simulink model "F16ASYM_Controlled"  (R2015a)
settings: Solver=ode3  SolverMode=SingleTasking  StartTime=0.0  StopTime=inf  FixedStep=T_sim  RelTol=1e-3
InitFcn:
  | load('NN_c_weights_Last_stable.mat')
StopFcn:
  | Final_results
values from neighbouring files (symbols this model uses):
  a1 = fitresult.p1    [Stall_protection.m]
  alpha_map_eval = ones(size(M_eval))*NaN    [Auto_trim_aid.m]    (also in Autotrim_maps.mat = [nan nan 0.277598136245 0.119432432992 0.0579479097061 0.027)
  beta_map_eval = ones(size(M_eval))*NaN    [Auto_trim_aid.m]    (also in Autotrim_maps.mat = [nan nan -0.00151549403324 0.00117807579006 -0.0052086799721)
  C_L_0 = fitresult.p2    [Stall_protection.m]
  G_eval = NaN*ones(size(M_sq,2),size(H_sq,2))    [Stall_protection.m]
  H_sq = unique(sort(H_sq))    [Stall_protection.m]
  H_sq_autotrim = min( F_envelope.H_1g):2000:max(F_envelope.H_1g)    [Auto_trim_aid.m]    (also in Autotrim_maps.mat = [0 2000 4000 6000 8000 10000 12000 14000 16000 18000])
  K_b_q_extrap_ACC = K_b_q_extrap    [RUN_ME.m]
  K_b_q_extrap_AoA = K_b_q_extrap    [RUN_ME.m]
  M_sq = unique(sort(M_sq))    [Stall_protection.m]
  M_sq_autotrim = 0:0.1:max(F_envelope.M_1g)    [Auto_trim_aid.m]    (also in Autotrim_maps.mat = [0 0.1 0.2 0.3 0.4 0.5 0.6 0.7 0.8 0.9 1 1.1 ... (21 element)
  T_sim = 0.02    [RUN_ME.m]
  tau_q_extrap_ACC = tau_q_extrap    [RUN_ME.m]
  tau_q_extrap_AoA = tau_q_extrap    [RUN_ME.m]
  velocity = M_eval(I,J)*a    [Auto_trim_aid.m]
undefined symbols (not defined in the file or in its folder): ACCEL, B, Earth, fi_flag_Simulink, GYRO, H_sq_sche, k_B, K_b_ACC_extrap, K_b_AoA_extrap, latitude, longitude, m, m_B, M_sq_sche, Model_used_flag, rad, s, sigbuilder_block, Stall_curve, tau_ACC_extrap, tau_AoA_extrap, Theta_1_roll_last, Theta_2_roll_last, Theta_3_roll_last, trim_control, trim_state, trim_throttle, V_Comp_A_w_z_last, V_Comp_last, V_Comp_last_ONE, V_long_lastA_w_z, V_long_lastAoA, V_roll_last, V_roll_lastMOD, V_yaw_last, W_Comp_A_w_z_last, W_Comp_last, W_long_lastA_w_z, W_long_lastAoA, W_roll_last, W_roll_lastMOD, W_yaw_last, WGS84
libraries: Adaptive_FaultTolerantControl x57, dspsigops x37, F16_Actuator_Library x14, commnoisgen2 x13, simulink x11, simulink_extras x10, dsparch4 x6, aerolibatmos2 x6, aerolibtransform2 x6, aerolibfltsims x3, dspvision x3, dspsnks4 x3
(part 6 of 14)

== system F16ASYM_Controlled/Primary Controller/P cont + adaptive Crossed NN + AWU+Lim ONELAYER/Physical limitation ==
  note: Converto to Angular accelerations
  v comm : Inport
  all meas : Inport  Port=2
  Ang Accel : MATLAB Function
  Bus Selector : BusSelector  OutputSignals=signal1.Alt meas (m),signal1.V_TAS (m/s),signal1.AoA meas (rad),signal1.SS meas (rad),signal1.omega_b meas (rad/s),signal1.Throttle_meas
  Bus Selector1 : BusSelector  OutputSignals=signal2.q (Pa),signal1.omega_b meas (rad/s)
  Demux : Demux  Outputs=3
  Display : Display
  Display1 : Display
  Display2 : Display
  Divide : Product  Inputs=**
  Divide1 : Product  Inputs=**
  Gain : Gain  Gain=-1
  Gain1 : Gain
  Mom coefficients that can be reached : MATLABFcn  MATLABFcn=Moms_Coeff_estimator  OutputDimensions=3  OutputSignalType=real
  Moments : Subsystem
  Mux : Mux  Inputs=3
  Mux1 : Mux  Inputs=7
  Saturation Dynamic : simulink/Discontinuities/Saturation Dynamic  OutMin=[]  OutMax=[]  OutDataTypeStr=Inherit: Same as second input  OutDataType=fixdt(1, 16)  OutScaling=2^-10  DoSatur=off
  Sign : Signum
  Sign1 : Signum
  max deflections estimator : MATLAB Function  TreatAsAtomicUnit=on
  v limted : Outport
  wires:
  max deflections estimator/1(max_defl) -> Mux1/7
  Mux1/1 -> Mom coefficients that can be reached/1
  Bus Selector/5 -> Mux1/5  "<omega_b meas (rad/s)>"
  Bus Selector/1 -> Mux1/1  "<Alt meas (m)>"
  Bus Selector/2 -> Mux1/2  "<V_TAS (m/s)>"
  Bus Selector/3 -> Mux1/3  "<AoA meas (rad)>"
  Bus Selector/4 -> Mux1/4  "<SS meas (rad)>"
  Bus Selector/6 -> Mux1/6  "<Throttle_meas>"
  Ang Accel/2(q_dot) -> Mux/2
  Ang Accel/3(r_dot) -> Mux/3
  Ang Accel/1(p_dot) -> Mux/1
  Bus Selector1/2 -> Ang Accel/4(omega_b)  "<omega_b meas (rad/s)>"
  Moments/3(N) -> Ang Accel/3(N)
  Moments/2(M) -> Ang Accel/2(M)
  Moments/1(L) -> Ang Accel/1(L)
  Bus Selector1/1 -> Moments/4(q)  "<q (Pa)>"
  Demux/3 -> Moments/3(C_N)
  Demux/2 -> Moments/2(C_M)
  Demux/1 -> Moments/1(C_L)
  Mom coefficients that can be reached/1 -> Demux/1
  all meas/1 -> Bus Selector/1, Bus Selector1/1
  Mux/1 -> Gain1/1
  v comm/1 -> Saturation Dynamic/2, Display1/1, max deflections estimator/1(v_comm)
  Saturation Dynamic/1 -> Display/1, v limted/1
  Sign/1 -> Divide/1
  Gain1/1 -> Divide/2, Divide1/1, Sign1/1, Display2/1, Sign/1
  Sign1/1 -> Gain/1
  Divide/1 -> Saturation Dynamic/1
  Gain/1 -> Divide1/2
  Divide1/1 -> Saturation Dynamic/3

== system F16ASYM_Controlled/Primary Controller/P cont + adaptive Crossed NN + AWU+Lim ONELAYER/Sigmoid  ==
  In : Inport
  Display : Display
  Fcn1 : Fcn  Commented=on  Expr=2.0 ./ (1.0 + exp(-u(4)*u(1:3)))-1
  MATLAB Function : MATLAB Function  TreatAsAtomicUnit=on
  a : Constant  Value=a
  Out : Outport
  wires:
  MATLAB Function/1(y) -> Display/1, Out/1
  In/1 -> MATLAB Function/1(u)
  a/1 -> MATLAB Function/2(a)

== system F16ASYM_Controlled/Primary Controller/P controller/Body Rates Controller ==
  p_ref : Inport
  q_ref : Inport  Port=2
  r_ref : Inport  Port=3
  All_meas : Inport  Port=4
  Bus Creator : BusCreator
  Bus Creator1 : BusCreator
  Bus Creator2 : BusCreator
  Bus Selector : BusSelector  OutputSignals=signal1.omega_b meas (rad/s)
  Display1 : Display
  Mux : Mux  Inputs=3
  Ref Model and P Controller p : Adaptive_FaultTolerantControl/Ref Model and P Controller  tau=0.1  y_i=trim_state(10)  K_f=1  K_b=7
  Ref Model and P Controller q : Adaptive_FaultTolerantControl/Ref Model and P Controller  tau=0.08  y_i=trim_state(11)  K_f=1  K_b=3.5
  Ref Model and P Controller r : Adaptive_FaultTolerantControl/Ref Model and P Controller  tau=0.08  y_i=trim_state(12)  K_f=1  K_b=4
  Selector : Selector  InputPortWidth=3
  Selector1 : Selector  InputPortWidth=3  Indices=2
  Selector2 : Selector  InputPortWidth=3  Indices=3
  Sum : Sum  Inputs=+-|
  Sum1 : Sum  Inputs=+-|
  Sum2 : Sum  Inputs=+-|
  Terminator1 : Terminator
  Terminator2 : Terminator
  Terminator3 : Terminator
  Angular acc des (rad/s^2) : Outport
  wires:
  Ref Model and P Controller r/5 -> Bus Creator2/4  "K_b_r"
  Ref Model and P Controller r/4 -> Sum2/2
  Sum2/1 -> Bus Creator2/3  "p_err"
  Ref Model and P Controller r/3 -> Bus Creator2/2, Sum2/1  "p_sf"
  Ref Model and P Controller r/2 -> Bus Creator2/1  "p_sf_dot"
  Ref Model and P Controller q/5 -> Bus Creator1/4  "K_b_q"
  Ref Model and P Controller q/4 -> Sum1/2
  Sum1/1 -> Bus Creator1/3  "p_err"
  Ref Model and P Controller q/3 -> Bus Creator1/2, Sum1/1  "p_sf"
  Ref Model and P Controller q/2 -> Bus Creator1/1  "p_sf_dot"
  Ref Model and P Controller p/5 -> Bus Creator/4  "K_b_p"
  Ref Model and P Controller p/4 -> Sum/2
  Selector2/1 -> Ref Model and P Controller r/2
  Bus Creator2/1 -> Terminator3/1
  Bus Creator1/1 -> Terminator1/1
  Bus Creator/1 -> Terminator2/1
  Sum/1 -> Bus Creator/3, Display1/1  "p_err"
  Ref Model and P Controller p/3 -> Bus Creator/2, Sum/1  "p_sf"
  Ref Model and P Controller p/2 -> Bus Creator/1  "p_sf_dot"
  Ref Model and P Controller r/1 -> Mux/3
  Ref Model and P Controller q/1 -> Mux/2
  r_ref/1 -> Ref Model and P Controller r/1
  Selector1/1 -> Ref Model and P Controller q/2
  q_ref/1 -> Ref Model and P Controller q/1
  Mux/1 -> Angular acc des (rad/s^2)/1
  Ref Model and P Controller p/1 -> Mux/1
  Selector/1 -> Ref Model and P Controller p/2
  p_ref/1 -> Ref Model and P Controller p/1
  Bus Selector/1 -> Selector2/1, Selector1/1, Selector/1  "<omega_b meas (rad/s)>"
  All_meas/1 -> Bus Selector/1

== system F16ASYM_Controlled/Primary Controller/P controller/Lat_dir Dyn Inversion: beta_dot->r_c ==
  beta_dot_c : Inport
  All_meas : Inport  Port=2
  A_w_y : Selector  InputPortWidth=3  Indices=2
  Bus Selector : BusSelector  OutputSignals=signal1.AoA meas (rad),signal1.omega_b meas (rad/s),signal1.V_TAS (m/s),signal2.A_w_CG
  Divide1 : Product  Inputs=**
  Divide3 : Product  Inputs=**
  Divide4 : Product  Inputs=/*
  Divide5 : Product  Inputs=*/
  Selector : Selector  InputPortWidth=3
  Trigonometric Function : Trigonometry  Operator=cos
  Trigonometric Function3 : Trigonometry  Operator=tan
  "q_c " : Sum  Inputs=-++
  r_c : Outport
  wires:
  Selector/1 -> Divide1/2
  Trigonometric Function3/1 -> Divide1/1
  beta_dot_c/1 -> Divide5/1
  Divide5/1 -> "q_c "/1
  Trigonometric Function/1 -> Divide5/2, Divide3/1
  Bus Selector/3 -> Divide3/2  "<V_TAS (m/s)>"
  Divide4/1 -> "q_c "/3
  Bus Selector/4 -> A_w_y/1  "<A_w_CG>"
  All_meas/1 -> Bus Selector/1
  A_w_y/1 -> Divide4/2
  Divide3/1 -> Divide4/1
  Divide1/1 -> "q_c "/2
  Bus Selector/2 -> Selector/1  "<omega_b meas (rad/s)>"
  Bus Selector/1 -> Trigonometric Function3/1, Trigonometric Function/1  "<AoA meas (rad)>"
  "q_c "/1 -> r_c/1

== system F16ASYM_Controlled/Primary Controller/P controller/Long Dyn Inversion: alpha_dot ->q ==
  alpha_dot_c : Inport
  All_meas : Inport  Port=2
  Completed : Subsystem
  Manual Switch : ManualSwitch
  Simplified : Subsystem
  q_c : Outport
  wires:
  Manual Switch/1 -> q_c/1
  Simplified/1(q_c) -> Manual Switch/2
  Completed/1(q_c) -> Manual Switch/1
  All_meas/1 -> Completed/2(All_meas), Simplified/2(All_meas)
  alpha_dot_c/1 -> Completed/1(alpha_dot_c), Simplified/1(alpha_dot_c)

== system F16ASYM_Controlled/Primary Controller/P controller/Longitudinal Controller: AoA or A_w_z ==
  A_w_z des : Inport
  AoA des (rad) : Inport  Port=2
  Anti-windup A_w_z : Inport  Port=3
  Anti-windup AoA : Inport  Port=4
  All meas : Inport  Port=5
  Longitudinal controller in A_w_z : Subsystem  VariantControl=Controller of A_w_z
  Longitudinal controller in AoA : Subsystem  VariantControl=Controller of AoA
  A_chanel vars : Outport
  alpha_chanel vars : Outport  Port=2
  alpha_dot_c : Outport  Port=3

== system F16ASYM_Controlled/Primary Controller/P controller + adaptive Crossed NN/Body Rates Controller ==
  p_ref : Inport
  q_ref : Inport  Port=2
  r_ref : Inport  Port=3
  All_meas : Inport  Port=4
  Bus Creator : BusCreator
  Bus Creator1 : BusCreator
  Bus Creator2 : BusCreator
  Bus Selector : BusSelector  OutputSignals=signal1.omega_b meas (rad/s)
  Display1 : Display
  Mux : Mux  Inputs=3
  Ref Model and P Controller p : Adaptive_FaultTolerantControl/Ref Model and P Controller  tau=0.1  y_i=trim_state(10)  K_f=1  K_b=7
  Ref Model and P Controller q : Adaptive_FaultTolerantControl/Ref Model and P Controller  tau=0.25  y_i=trim_state(11)  K_f=1  K_b=7
  Ref Model and P Controller r : Adaptive_FaultTolerantControl/Ref Model and P Controller  tau=0.2  y_i=trim_state(12)  K_f=1  K_b=4
  Selector : Selector  InputPortWidth=3
  Selector1 : Selector  InputPortWidth=3  Indices=2
  Selector2 : Selector  InputPortWidth=3  Indices=3
  Sum : Sum  Inputs=+-|
  Sum1 : Sum  Inputs=+-|
  Sum2 : Sum  Inputs=+-|
  q_chanel vars : Outport
  p_chanel vars : Outport  Port=2
  r_chanel vars : Outport  Port=3
  Angular acc des (rad/s^2) : Outport  Port=4
  wires:
  Ref Model and P Controller r/5 -> Bus Creator2/4  "K_b_r"
  Ref Model and P Controller r/4 -> Sum2/2
  Sum2/1 -> Bus Creator2/3  "r_err"
  Ref Model and P Controller r/3 -> Bus Creator2/2, Sum2/1  "r_sf"
  Ref Model and P Controller r/2 -> Bus Creator2/1  "r_sf_dot"
  Ref Model and P Controller q/5 -> Bus Creator1/4  "K_b_q"
  Ref Model and P Controller q/4 -> Sum1/2
  Sum1/1 -> Bus Creator1/3  "q_err"
  Ref Model and P Controller q/3 -> Bus Creator1/2, Sum1/1  "q_sf"
  Ref Model and P Controller q/2 -> Bus Creator1/1  "q_sf_dot"
  Ref Model and P Controller p/5 -> Bus Creator/4  "K_b_p"
  Ref Model and P Controller p/4 -> Sum/2
  Selector2/1 -> Ref Model and P Controller r/2
  Bus Creator2/1 -> r_chanel vars/1
  Bus Creator1/1 -> q_chanel vars/1
  Bus Creator/1 -> p_chanel vars/1
  Sum/1 -> Bus Creator/3, Display1/1  "p_err"
  Ref Model and P Controller p/3 -> Bus Creator/2, Sum/1  "p_sf"
  Ref Model and P Controller p/2 -> Bus Creator/1  "p_sf_dot"
  Ref Model and P Controller r/1 -> Mux/3
  Ref Model and P Controller q/1 -> Mux/2
  r_ref/1 -> Ref Model and P Controller r/1
  Selector1/1 -> Ref Model and P Controller q/2
  q_ref/1 -> Ref Model and P Controller q/1
  Mux/1 -> Angular acc des (rad/s^2)/1
  Ref Model and P Controller p/1 -> Mux/1
  Selector/1 -> Ref Model and P Controller p/2
  p_ref/1 -> Ref Model and P Controller p/1
  Bus Selector/1 -> Selector2/1, Selector1/1, Selector/1  "<omega_b meas (rad/s)>"
  All_meas/1 -> Bus Selector/1

== system F16ASYM_Controlled/Primary Controller/P controller + adaptive Crossed NN/Complete crossed On-line (adaptive) multi-layer NN ==
  v_ad^ prev : Inport
  All_meas : Inport  Port=2
  NN variables : Inport  Port=3
  Complete crossed On-line (adaptive) multi-layer NN: A_w_z : Subsystem  VariantControl=NN on A_w_z
  Complete crossed On-line (adaptive) multi-layer NN: AoA : Subsystem  VariantControl=NN on AoA
  v_ad^ : Outport

== system F16ASYM_Controlled/Primary Controller/P controller + adaptive Crossed NN/Lat_dir Dyn Inversion: beta_dot->r_c ==
  beta_dot_c : Inport
  All_meas : Inport  Port=2
  A_w_y : Selector  InputPortWidth=3  Indices=2
  Bus Selector : BusSelector  OutputSignals=signal1.AoA meas (rad),signal1.omega_b meas (rad/s),signal1.V_TAS (m/s),signal2.A_w_CG
  Divide1 : Product  Inputs=**
  Divide3 : Product  Inputs=**
  Divide4 : Product  Inputs=/*
  Divide5 : Product  Inputs=*/
  Selector : Selector  InputPortWidth=3
  Trigonometric Function : Trigonometry  Operator=cos
  Trigonometric Function3 : Trigonometry  Operator=tan
  "q_c " : Sum  Inputs=-++
  r_c : Outport
  wires:
  Selector/1 -> Divide1/2
  Trigonometric Function3/1 -> Divide1/1
  beta_dot_c/1 -> Divide5/1
  Divide5/1 -> "q_c "/1
  Trigonometric Function/1 -> Divide5/2, Divide3/1
  Bus Selector/3 -> Divide3/2  "<V_TAS (m/s)>"
  Divide4/1 -> "q_c "/3
  Bus Selector/4 -> A_w_y/1  "<A_w_CG>"
  All_meas/1 -> Bus Selector/1
  A_w_y/1 -> Divide4/2
  Divide3/1 -> Divide4/1
  Divide1/1 -> "q_c "/2
  Bus Selector/2 -> Selector/1  "<omega_b meas (rad/s)>"
  Bus Selector/1 -> Trigonometric Function3/1, Trigonometric Function/1  "<AoA meas (rad)>"
  "q_c "/1 -> r_c/1

== system F16ASYM_Controlled/Primary Controller/P controller + adaptive Crossed NN/Long Dyn Inversion: alpha_dot ->q ==
  alpha_dot_c : Inport
  All_meas : Inport  Port=2
  Completed : Subsystem
  Manual Switch : ManualSwitch
  Simplified : Subsystem
  q_c : Outport
  wires:
  Manual Switch/1 -> q_c/1
  Simplified/1(q_c) -> Manual Switch/2
  Completed/1(q_c) -> Manual Switch/1
  All_meas/1 -> Completed/2(All_meas), Simplified/2(All_meas)
  alpha_dot_c/1 -> Completed/1(alpha_dot_c), Simplified/1(alpha_dot_c)

== system F16ASYM_Controlled/Primary Controller/P controller + adaptive Crossed NN/Longitudinal Controller: AoA or A_w_z ==
  A_w_z des : Inport
  AoA des (rad) : Inport  Port=2
  Anti-windup A_w_z : Inport  Port=3
  Anti-windup AoA : Inport  Port=4
  All meas : Inport  Port=5
  Longitudinal controller in A_w_z : Subsystem  VariantControl=Controller of A_w_z
  Longitudinal controller in AoA : Subsystem  VariantControl=Controller of AoA
  A_chanel vars : Outport
  alpha_chanel vars : Outport  Port=2
  alpha_dot_c : Outport  Port=3

== system F16ASYM_Controlled/Primary Controller/P controller + adaptive Crossed NN/Sigmoid  ==
  In : Inport
  Display : Display
  Fcn1 : Fcn  Commented=on  Expr=2.0 ./ (1.0 + exp(-u(4)*u(1:3)))-1
  MATLAB Function : MATLAB Function  TreatAsAtomicUnit=on
  a : Constant  Value=a
  Out : Outport
  wires:
  a/1 -> MATLAB Function/2(a)
  In/1 -> MATLAB Function/1(u)
  MATLAB Function/1(y) -> Out/1, Display/1

== system F16ASYM_Controlled/Primary Controller/P controller + adaptive Isolated NN/Body Rates Controller ==
  p_ref : Inport
  q_ref : Inport  Port=2
  r_ref : Inport  Port=3
  All_meas : Inport  Port=4
  Bus Creator : BusCreator
  Bus Creator1 : BusCreator
  Bus Creator2 : BusCreator
  Bus Selector : BusSelector  OutputSignals=signal1.omega_b meas (rad/s)
  Display1 : Display
  Mux : Mux  Inputs=3
  Ref Model and P Controller p : Adaptive_FaultTolerantControl/Ref Model and P Controller  tau=0.1  y_i=trim_state(10)  K_f=1  K_b=7
  Ref Model and P Controller q : Adaptive_FaultTolerantControl/Ref Model and P Controller  tau=0.25  y_i=trim_state(11)  K_f=1  K_b=8
  Ref Model and P Controller r : Adaptive_FaultTolerantControl/Ref Model and P Controller  tau=0.2  y_i=trim_state(12)  K_f=1  K_b=4
  Selector : Selector  InputPortWidth=3
  Selector1 : Selector  InputPortWidth=3  Indices=2
  Selector2 : Selector  InputPortWidth=3  Indices=3
  Sum : Sum  Inputs=+-|
  Sum1 : Sum  Inputs=+-|
  Sum2 : Sum  Inputs=+-|
  q_chanel vars : Outport
  p_chanel vars : Outport  Port=2
  r_chanel vars : Outport  Port=3
  Angular acc des (rad/s^2) : Outport  Port=4
  wires:
  All_meas/1 -> Bus Selector/1
  Bus Selector/1 -> Selector/1, Selector1/1, Selector2/1  "<omega_b meas (rad/s)>"
  p_ref/1 -> Ref Model and P Controller p/1
  Selector/1 -> Ref Model and P Controller p/2
  Ref Model and P Controller p/1 -> Mux/1
  Mux/1 -> Angular acc des (rad/s^2)/1
  q_ref/1 -> Ref Model and P Controller q/1
  Selector1/1 -> Ref Model and P Controller q/2
  r_ref/1 -> Ref Model and P Controller r/1
  Ref Model and P Controller q/1 -> Mux/2
  Ref Model and P Controller r/1 -> Mux/3
  Ref Model and P Controller p/2 -> Bus Creator/1  "p_sf_dot"
  Ref Model and P Controller p/3 -> Sum/1, Bus Creator/2  "p_sf"
  Sum/1 -> Display1/1, Bus Creator/3  "p_err"
  Bus Creator/1 -> p_chanel vars/1
  Bus Creator1/1 -> q_chanel vars/1
  Bus Creator2/1 -> r_chanel vars/1
  Selector2/1 -> Ref Model and P Controller r/2
  Ref Model and P Controller p/4 -> Sum/2
  Ref Model and P Controller p/5 -> Bus Creator/4  "K_b_p"
  Ref Model and P Controller q/2 -> Bus Creator1/1  "q_sf_dot"
  Ref Model and P Controller q/3 -> Sum1/1, Bus Creator1/2  "q_sf"
  Sum1/1 -> Bus Creator1/3  "q_err"
  Ref Model and P Controller q/4 -> Sum1/2
  Ref Model and P Controller q/5 -> Bus Creator1/4  "K_b_q"
  Ref Model and P Controller r/2 -> Bus Creator2/1  "r_sf_dot"
  Ref Model and P Controller r/3 -> Sum2/1, Bus Creator2/2  "r_sf"
  Sum2/1 -> Bus Creator2/3  "r_err"
  Ref Model and P Controller r/4 -> Sum2/2
  Ref Model and P Controller r/5 -> Bus Creator2/4  "K_b_r"

== system F16ASYM_Controlled/Primary Controller/P controller + adaptive Isolated NN/Lat_dir Dyn Inversion: beta_dot->r_c ==
  beta_dot_c : Inport
  All_meas : Inport  Port=2
  A_w_y : Selector  InputPortWidth=3  Indices=2
  Bus Selector : BusSelector  OutputSignals=signal1.AoA meas (rad),signal1.omega_b meas (rad/s),signal1.V_TAS (m/s),signal2.A_w_CG
  Divide1 : Product  Inputs=**
  Divide3 : Product  Inputs=**
  Divide4 : Product  Inputs=/*
  Divide5 : Product  Inputs=*/
  Selector : Selector  InputPortWidth=3
  Trigonometric Function : Trigonometry  Operator=cos
  Trigonometric Function3 : Trigonometry  Operator=tan
  "q_c " : Sum  Inputs=-++
  r_c : Outport
  wires:
  "q_c "/1 -> r_c/1
  Bus Selector/1 -> Trigonometric Function/1, Trigonometric Function3/1  "<AoA meas (rad)>"
  Bus Selector/2 -> Selector/1  "<omega_b meas (rad/s)>"
  Divide1/1 -> "q_c "/2
  Divide3/1 -> Divide4/1
  A_w_y/1 -> Divide4/2
  All_meas/1 -> Bus Selector/1
  Bus Selector/4 -> A_w_y/1  "<A_w_CG>"
  Divide4/1 -> "q_c "/3
  Bus Selector/3 -> Divide3/2  "<V_TAS (m/s)>"
  Trigonometric Function/1 -> Divide3/1, Divide5/2
  Divide5/1 -> "q_c "/1
  beta_dot_c/1 -> Divide5/1
  Trigonometric Function3/1 -> Divide1/1
  Selector/1 -> Divide1/2

== system F16ASYM_Controlled/Primary Controller/P controller + adaptive Isolated NN/Long Dyn Inversion: alpha_dot ->q ==
  alpha_dot_c : Inport
  All_meas : Inport  Port=2
  Completed : Subsystem
  Manual Switch : ManualSwitch
  Simplified : Subsystem
  q_c : Outport
  wires:
  alpha_dot_c/1 -> Simplified/1(alpha_dot_c), Completed/1(alpha_dot_c)
  All_meas/1 -> Simplified/2(All_meas), Completed/2(All_meas)
  Completed/1(q_c) -> Manual Switch/1
  Simplified/1(q_c) -> Manual Switch/2
  Manual Switch/1 -> q_c/1

== system F16ASYM_Controlled/Primary Controller/P controller + adaptive Isolated NN/Longitudinal Controller: AoA or A_w_z ==
  A_w_z des : Inport
  AoA des (rad) : Inport  Port=2
  Anti-windup A_w_z : Inport  Port=3
  Anti-windup AoA : Inport  Port=4
  All meas : Inport  Port=5
  Longitudinal controller in A_w_z : Subsystem  VariantControl=Controller of A_w_z
  Longitudinal controller in AoA : Subsystem  VariantControl=Controller of AoA
  A_chanel vars : Outport
  alpha_chanel vars : Outport  Port=2
  alpha_dot_c : Outport  Port=3

== system F16ASYM_Controlled/Primary Controller/P controller + adaptive Isolated NN/On-line (adaptive) multi-layer NNs ==
  v_ad^ prev : Inport
  All_meas : Inport  Port=2
  NN variables : Inport  Port=3
  Bus Selector : BusSelector  OutputSignals=p_chanel_vars,Long chanel,beta_r_chanel
  Long Chanel : Subsystem  Variant=on  OverrideUsingVariant=Long HL NN A_w_z
  Long_learning rate : Constant  Value=30.5  SampleTime=T_sim
  Long_reg param : Constant  SampleTime=T_sim
  Mux : Mux  Inputs=3
  Roll NN : Subsystem  Variant=on  OverrideUsingVariant=Roll 2HL NN
  Roll_learning rate : Constant  Value=73  SampleTime=T_sim
  Roll_reg param : Constant  SampleTime=T_sim
  Selector : Selector  InputPortWidth=3
  Selector1 : Selector  InputPortWidth=3  Indices=2
  Selector2 : Selector  InputPortWidth=3  Indices=3
  Yaw Chanel : Subsystem  Variant=on  OverrideUsingVariant=Yaw HL NN
  Yaw_learning rate : Constant  Value=20.8  SampleTime=T_sim
  Yaw_reg param : Constant  Value=0.8  SampleTime=T_sim
  v_ad^ prev1 : InportShadow
  v_ad^ prev2 : InportShadow
  v_ad^ : Outport
  wires:
  NN variables/1 -> Bus Selector/1
  Bus Selector/1 -> Roll NN/2(p_chanel vars)  "<p_chanel_vars>"
  All_meas/1 -> Yaw Chanel/3(All_meas), Long Chanel/3(All_meas), Roll NN/3(All_meas)
  Roll NN/1(v_ad_comp) -> Mux/1
  Mux/1 -> v_ad^/1
  v_ad^ prev/1 -> Selector/1
  Selector/1 -> Roll NN/1(v_ad^ prev)
  Roll_learning rate/1 -> Roll NN/4(Roll_learning rate)
  Roll_reg param/1 -> Roll NN/5(Roll reg param)
  Selector1/1 -> Long Chanel/1(v_ad^ prev)
  Long_learning rate/1 -> Long Chanel/4(Long_learning rate)
  Long_reg param/1 -> Long Chanel/5(Long reg param)
  v_ad^ prev1/1 -> Selector1/1
  Bus Selector/2 -> Long Chanel/2(Long_chanel vars)  "<Long chanel>"
  Yaw_learning rate/1 -> Yaw Chanel/4(Yaw_learning rate)
  Yaw_reg param/1 -> Yaw Chanel/5(Yaw reg param)
  v_ad^ prev2/1 -> Selector2/1
  Selector2/1 -> Yaw Chanel/1(v_ad^ prev)
  Bus Selector/3 -> Yaw Chanel/2(Yaw_chanel vars)  "<beta_r_chanel>"
  Yaw Chanel/1(v_ad_comp) -> Mux/3
  Long Chanel/1(v_ad_comp) -> Mux/2

== system F16ASYM_Controlled/Primary Controller/P controller + adaptive Isolated NN/On-line (adaptive) multi-layer NNs SIMPL ==
  v_ad^ prev : Inport
  All_meas : Inport  Port=2
  NN variables : Inport  Port=3
  Bus Selector : BusSelector  OutputSignals=p_chanel_vars,Long chanel,beta_r_chanel
  Long Chanel : Subsystem  Variant=on  OverrideUsingVariant=Long HL NN A_w_z
  Long_learning rate : Constant  Value=19.7  SampleTime=T_sim
  Long_reg param : Constant  Value=0.9  SampleTime=T_sim
  Mux : Mux  Inputs=3
  Roll NN : Subsystem  Variant=on  OverrideUsingVariant=Roll 1HL NN
  Roll_learning rate : Constant  Value=80  SampleTime=T_sim
  Roll_reg param : Constant  Value=0.5  SampleTime=T_sim
  Selector : Selector  InputPortWidth=3
  Selector1 : Selector  InputPortWidth=3  Indices=2
  Selector2 : Selector  InputPortWidth=3  Indices=3
  Yaw Chanel : Subsystem  Variant=on  OverrideUsingVariant=Yaw HL NN
  Yaw_learning rate : Constant  Value=20.5  SampleTime=T_sim
  Yaw_reg param : Constant  SampleTime=T_sim
  v_ad^ prev1 : InportShadow
  v_ad^ prev2 : InportShadow
  v_ad^ : Outport
  wires:
  Long Chanel/1(v_ad_comp) -> Mux/2
  Yaw Chanel/1(v_ad_comp) -> Mux/3
  Bus Selector/3 -> Yaw Chanel/2(Yaw_chanel vars)  "<beta_r_chanel>"
  Selector2/1 -> Yaw Chanel/1(v_ad^ prev)
  v_ad^ prev2/1 -> Selector2/1
  Yaw_reg param/1 -> Yaw Chanel/5(Yaw reg param)
  Yaw_learning rate/1 -> Yaw Chanel/4(Yaw_learning rate)
  Bus Selector/2 -> Long Chanel/2(Long_chanel vars)  "<Long chanel>"
  v_ad^ prev1/1 -> Selector1/1
  Long_reg param/1 -> Long Chanel/5(Long reg param)
  Long_learning rate/1 -> Long Chanel/4(Long_learning rate)
  Selector1/1 -> Long Chanel/1(v_ad^ prev)
  Roll_reg param/1 -> Roll NN/5(Roll reg param)
  Roll_learning rate/1 -> Roll NN/4(Roll_learning rate)
  Selector/1 -> Roll NN/1(v_ad^ prev)
  v_ad^ prev/1 -> Selector/1
  Mux/1 -> v_ad^/1
  Roll NN/1(v_ad_comp) -> Mux/1
  All_meas/1 -> Roll NN/3(All_meas), Long Chanel/3(All_meas), Yaw Chanel/3(All_meas)
  Bus Selector/1 -> Roll NN/2(p_chanel vars)  "<p_chanel_vars>"
  NN variables/1 -> Bus Selector/1

== system F16ASYM_Controlled/Primary Controller/P controller + adaptive Isolated NN/Sigmoid  ==
  In : Inport
  Display : Display
  Fcn1 : Fcn  Commented=on  Expr=2.0 ./ (1.0 + exp(-u(4)*u(1:3)))-1
  MATLAB Function : MATLAB Function  TreatAsAtomicUnit=on
  a : Constant  Value=a
  Out : Outport
  wires:
  MATLAB Function/1(y) -> Display/1, Out/1
  In/1 -> MATLAB Function/1(u)
  a/1 -> MATLAB Function/2(a)

== system F16ASYM_Controlled/Primary Controller/PI Primary Controller/Body Rates Controller ==
  p_ref : Inport
  q_ref : Inport  Port=2
  r_ref : Inport  Port=3
  All_meas : Inport  Port=4
  All Anti-windup signals : Inport  Port=5
  Bus Creator : BusCreator  Inputs=3
  Bus Creator1 : BusCreator  Inputs=3
  Bus Creator2 : BusCreator  Inputs=3
  Bus Selector : BusSelector  OutputSignals=signal1.omega_b meas (rad/s)
  Display : Display
  Mux : Mux  Inputs=3
  Ref Model and PI Controller P : Adaptive_FaultTolerantControl/Ref Model and PI Controller  delta=0  tau=0.2  y_i=trim_state(10)  K_f=0.8  K_a=3  Con_way=pro  omega_n=4  xi=0.5  Z1=-30  K_b=10  f_i=0.2  f_c=1
  Ref Model and PI Controller q : Adaptive_FaultTolerantControl/Ref Model and PI Controller  delta=trim_state(11)  tau=0.15  y_i=0  K_f=0.8  K_a=3  Con_way=pro  omega_n=4  xi=0.5  Z1=-30  K_b=5  f_i=0.1  f_c=1
  Ref Model and PI Controller r : Adaptive_FaultTolerantControl/Ref Model and PI Controller  delta=trim_state(12)  tau=0.2  y_i=0  K_f=0.8  K_a=3  Con_way=pro  omega_n=4  xi=0.5  Z1=-30  K_b=10  f_i=0.2  f_c=1
  Selector : Selector  InputPortWidth=3
  Selector1 : Selector  InputPortWidth=3  Indices=2
  Selector2 : Selector  InputPortWidth=3  Indices=3
  Selector3 : Selector  InputPortWidth=3
  Selector4 : Selector  InputPortWidth=3  Indices=2
  Selector5 : Selector  InputPortWidth=3  Indices=3
  Sum : Sum  Inputs=|+-
  Sum1 : Sum  Inputs=|+-
  Sum2 : Sum  Inputs=|+-
  Terminator : Terminator
  Terminator1 : Terminator
  Terminator2 : Terminator
  Angular acc des (rad/s^2) : Outport
  wires:
  Bus Creator2/1 -> Terminator2/1
  Sum2/1 -> Bus Creator2/3  "r_err"
  Ref Model and PI Controller r/4 -> Sum2/2
  Ref Model and PI Controller r/3 -> Bus Creator2/2, Sum2/1  "r_sf"
  Ref Model and PI Controller r/2 -> Bus Creator2/1  "r_sf_dot"
  Bus Creator1/1 -> Terminator1/1
  Sum1/1 -> Bus Creator1/3  "q_err"
  Ref Model and PI Controller q/4 -> Sum1/2
  Ref Model and PI Controller q/3 -> Bus Creator1/2, Sum1/1  "q_sf"
  Ref Model and PI Controller q/2 -> Bus Creator1/1  "q_sf_dot"
  Bus Creator/1 -> Terminator/1
  Sum/1 -> Bus Creator/3  "p_err"
  Ref Model and PI Controller P/4 -> Sum/2
  Ref Model and PI Controller P/3 -> Bus Creator/2, Sum/1  "p_sf"
  Ref Model and PI Controller P/2 -> Bus Creator/1  "p_sf_dot"
  Selector3/1 -> Ref Model and PI Controller P/3
  Selector5/1 -> Ref Model and PI Controller r/3
  Selector4/1 -> Ref Model and PI Controller q/3, Display/1
  All Anti-windup signals/1 -> Selector3/1, Selector5/1, Selector4/1
  Ref Model and PI Controller r/1 -> Mux/3
  Ref Model and PI Controller q/1 -> Mux/2
  r_ref/1 -> Ref Model and PI Controller r/1
  Selector2/1 -> Ref Model and PI Controller r/2
  Selector1/1 -> Ref Model and PI Controller q/2
  q_ref/1 -> Ref Model and PI Controller q/1
  Mux/1 -> Angular acc des (rad/s^2)/1
  Ref Model and PI Controller P/1 -> Mux/1
  Selector/1 -> Ref Model and PI Controller P/2
  p_ref/1 -> Ref Model and PI Controller P/1
  Bus Selector/1 -> Selector/1, Selector1/1, Selector2/1  "<omega_b meas (rad/s)>"
  All_meas/1 -> Bus Selector/1

== system F16ASYM_Controlled/Primary Controller/PI Primary Controller/Lat_dir Dyn Inversion: beta_dot->r_c ==
  beta_dot_c : Inport
  All_meas : Inport  Port=2
  A_w_y : Selector  InputPortWidth=3  Indices=2
  Bus Selector : BusSelector  OutputSignals=signal1.AoA meas (rad),signal1.omega_b meas (rad/s),signal1.V_TAS (m/s),signal2.A_w_CG
  Divide1 : Product  Inputs=**
  Divide3 : Product  Inputs=**
  Divide4 : Product  Inputs=/*
  Divide5 : Product  Inputs=*/
  Selector : Selector  InputPortWidth=3
  Trigonometric Function : Trigonometry  Operator=cos
  Trigonometric Function3 : Trigonometry  Operator=tan
  "q_c " : Sum  Inputs=-++
  r_c : Outport
  wires:
  Selector/1 -> Divide1/2
  Trigonometric Function3/1 -> Divide1/1
  beta_dot_c/1 -> Divide5/1
  Divide5/1 -> "q_c "/1
  Trigonometric Function/1 -> Divide5/2, Divide3/1
  Bus Selector/3 -> Divide3/2  "<V_TAS (m/s)>"
  Divide4/1 -> "q_c "/3
  Bus Selector/4 -> A_w_y/1  "<A_w_CG>"
  All_meas/1 -> Bus Selector/1
  A_w_y/1 -> Divide4/2
  Divide3/1 -> Divide4/1
  Divide1/1 -> "q_c "/2
  Bus Selector/2 -> Selector/1  "<omega_b meas (rad/s)>"
  Bus Selector/1 -> Trigonometric Function3/1, Trigonometric Function/1  "<AoA meas (rad)>"
  "q_c "/1 -> r_c/1

== system F16ASYM_Controlled/Primary Controller/PI Primary Controller/Long Dyn Inversion: alpha_dot ->q ==
  alpha_dot_c : Inport
  All_meas : Inport  Port=2
  Completed : Subsystem
  Manual Switch : ManualSwitch
  Simplified : Subsystem
  q_c : Outport
  wires:
  Manual Switch/1 -> q_c/1
  Simplified/1(q_c) -> Manual Switch/2
  Completed/1(q_c) -> Manual Switch/1
  All_meas/1 -> Completed/2(All_meas), Simplified/2(All_meas)
  alpha_dot_c/1 -> Completed/1(alpha_dot_c), Simplified/1(alpha_dot_c)

== system F16ASYM_Controlled/Primary Controller/PI Primary Controller/Longitudinal Controller: AoA or A_w_z ==
  A_w_z des : Inport
  AoA des (rad) : Inport  Port=2
  Anti-windup A_w_z : Inport  Port=3
  Anti-windup AoA : Inport  Port=4
  All meas : Inport  Port=5
  Longitudinal controller in A_w_z : Subsystem  VariantControl=Controller of A_w_z
  Longitudinal controller in AoA : Subsystem  VariantControl=Controller of AoA
  alpha_dot_c : Outport

== system F16ASYM_Controlled/SI and FDI/SI and FDI: Realistic/FDI: Assumed? ==
  note: Add noise, uncertainty and delay here!!!
  note: RECONFIGURATION PARAMETERS
      |
      | 24. mass  Estimated mass
      | 25. S_current_L
      | 26. S_current_R
      | 27. S_fin_current
      | 28. x_cg
      | 29. Jy
      | 30. Jxz
      | 31. Jz
      | 32. Jx
      | 33. EFF_el_L
      | 34. EFF_el_R
      | 35. EFF_ail_L
      | 36. EFF_ail_R
      | 37. EFF_rud
      | 38. EFF_lef_L
      | 39. EFF_lef_R
      | 40. Delta_C_Lift_X
      | 41. Delta_C_Drag_X
      | 42. Delta_C_m_X
  Inexistent Reconfig bus : Inport
  All  meas : Inport  Port=2
  Control comms : Inport  Port=3
  1st order model : Subsystem  mask{tau=0.3, y_i=ones(1,7)}
      mask prompts: tau "1st order time constant (tau)"; y_i "Initial state"
      mask init:
      | K_ref=1/tau;
      mask Display:
      | [y,t]=step(tf([K_ref],[1 K_ref]));
      | pos = get_param(gcb, 'Position');
      | width = pos(3) - pos(1);
      | height = pos(4) - pos(2);
      | t = t.*width/max(t);
      | y=y.*height/max(y);
      | plot(t,y);
      | 
      | 
      | text(0.5*width,0.92*height,['tau=',num2str(tau)]);
      | 
      | dpoly([K_ref],[1 K_ref], 's')
  Bus Selector : BusSelector  OutputSignals=Reconfig signal,Blockades,Blockade now
  Delay1 : Delay  DelayLength=floor(0.2/T_sim)  InitialCondition=NaN
  Delay2 : Delay  Commented=on  DelayLength=floor(0.2/T_sim)  InitialCondition=1
  Delay4 : Delay  DelayLength=floor(0.3/T_sim)  InitialCondition=0
  Delays : Subsystem
  Gaussian Noise Generator : commnoisgen2/Gaussian Noise Generator  m=0  d=0.00005*eye(7,7)  s=42  Ts=T_sim  frameBased=off  sampPerFrame=1  orient=off  outDataType=double
  ONLY Effectiveness : Selector  InputPortWidth=19  Indices=10:16
  Saturation : Saturate  UpperLimit=1  LowerLimit=0
  Scope1 : Scope
      settings: TimeRange=50  YMin=-20  YMax=10  SaveName=ScopeData12
  Scope2 : Scope  Commented=on
      settings: TimeRange=50  YMin=-17.5  YMax=17.5  SaveName=ScopeData26
  Scope3 : Scope
      settings: TimeRange=35  YMin=0.99525  YMax=1  SaveName=ScopeData39
  Sum : Sum  Inputs=++|
  Terminator : Terminator
  To Workspace : ToWorkspace  Commented=on  VariableName=FDI_effect_real  SaveFormat=Timeseries  SampleTime=-1
  To Workspace1 : ToWorkspace  VariableName=FDI_effect_fake  SaveFormat=Timeseries  SampleTime=-1
  To Workspace2 : ToWorkspace  Commented=on  VariableName=FDI_block_real  SaveFormat=Timeseries  SampleTime=-1
  To Workspace3 : ToWorkspace  VariableName=FDI_block_fake  SaveFormat=Timeseries  SampleTime=-1
  To Workspace4 : ToWorkspace  Commented=on  VariableName=FDI_control  SaveFormat=Timeseries  SampleTime=-1
  only deflections : Selector  InputPortWidth=8  Indices=2:8
  Blockades at : Outport
  Blockades now : Outport  Port=2
  Effectiveness : Outport  Port=3
  wires:
  Bus Selector/3 -> Delay4/1  "<Blockade now>"
  Bus Selector/2 -> To Workspace2/1, Delay1/1  "<Blockades>"
  Inexistent Reconfig bus/1 -> Bus Selector/1
  All  meas/1 -> Terminator/1
  ONLY Effectiveness/1 -> Sum/2, To Workspace/1
  Saturation/1 -> To Workspace1/1, Scope3/1, Effectiveness/1  "Effectiveness"
  Bus Selector/1 -> ONLY Effectiveness/1  "<Reconfig signal>"
  Delays/1(blockades at) -> To Workspace3/1, Scope1/1, Blockades at/1  "Blockades"
  Control comms/1 -> only deflections/1
  only deflections/1 -> Delays/2(Control comms), To Workspace4/1, Scope2/1
  Delay1/1 -> Delays/1(Blockades)
  Delay4/1 -> Blockades now/1  "Blockade now"
  Sum/1 -> 1st order model/1(y_in)
  1st order model/1(y_out) -> Saturation/1
  Gaussian Noise Generator/1 -> Sum/1

== system F16ASYM_Controlled/SI and FDI/SI and FDI: Realistic/SI ==
  note: Include here a logic that takes into account P so if the estimation is very bad do something
  note: Something to be done here!!!
  note: No estimation on this yet
  note: No estimation on this yet
  note: INPUTS
      | States:
      |
      | 1. Altitude
      | 2. TAS velocity
      | 3. alpha in rad
      | 4. beta in rads
      | 5. P
      | 6. Q
      | 7. R
      | 8. Throttle
      | 9. Elevator_L in deg
      | 10. Elevator_R in deg
      | 11. Aileron_L
      | 12. Aileron_R
      | 13. Rudder
      | 14. LEF_L
      | 15. LEF_R
      |
      | RECONFIGURATION PARAMETERS
      |
      | 16. mass  Estimated mass
      | 17. S_current_L
      | 18. S_current_R
      | 19. S_fin_current
      | 20. x_cg
      | 21. Jy
      | 22. Jxz
      | 23. Jz
      | 24. Jx
      | 25. EFF_el_L
      | 26. EFF_el_R
      | 27. EFF_ail_L
      | 28 EFF_ail_R
      | 29. EFF_rud
      | 30. EFF_lef_L
      | 31. EFF_lef_R
      | 32. Delta_C_Lift_X
      | 33. Delta_C_Drag_X
      | 34. Delta_C_m_X
  Control Eff : Inport
  All meas : Inport  Port=2
  Control comms : Inport  Port=3
  Base-line model parameters : Constant  Commented=on  Value=[9295.44,27.87/2,27.87/2,6.578,0.3,75673.6,1331.4,85552.1,12874.8]
  Bus Selector1 : BusSelector  OutputSignals=signal1.Alt meas (m),signal1.V_TAS (m/s),signal1.AoA meas (rad),signal1.SS meas (rad),signal1.omega_b meas (rad/s)
  Bus Selector2 : BusSelector  OutputSignals=signal1.omega_b meas (rad/s)
  Demux : Demux  Outputs=3
  Derivative : Derivative  CoefficientInTFapproximation=900
  Determinant of 3x3 Matrix : aerolibutil/Determinant of 3x3 Matrix
  Mass properties estimated : Constant  Value=[9295.44,0.3,75673.6,1331.4,85552.1,12874.8]
  Memory : Memory  X0=1*eye(3)
  Memory1 : Memory  X0=[27.87/2,27.87/2,6.578]
  Mux : Mux  Inputs=3
  Mux1 : Mux  Inputs=3
  NO-deviations from base-line model : Constant  Value=zeros(1,3)
  Scope : Scope
      settings: ShowLegends=on  TimeRange=50  YMin=6  YMax=14.5  SaveName=ScopeData23
  Scope1 : Scope
      settings: YMin=-1.75  YMax=2  SaveName=ScopeData24
  Scope2 : Scope
      settings: ShowLegends=on  TimeRange=50  YMin=15.05  YMax=16.15  SaveName=ScopeData2
  Surfaces UKF estimator : MATLAB Function  TreatAsAtomicUnit=on
  To Workspace : ToWorkspace  VariableName=SI_Surfaces_est  SaveFormat=Timeseries  SampleTime=-1
  To Workspace1 : ToWorkspace  VariableName=SI_P_matrix  SaveFormat=Timeseries  SampleTime=-1
  To Workspace2 : ToWorkspace  VariableName=SI_input  SaveFormat=Timeseries  SampleTime=-1
  f(x)  Mom Coefficients due to the dynamics: Coefficients model with control inputs : MATLABFcn  Commented=on  MATLABFcn=Moms_Coeff_Reconf_estimator  OutputDimensions=3  OutputSignalType=real
  Est Mass props : Outport
  Est Surfs : Outport  Port=2
  Est Aero changes : Outport  Port=3
  wires:
  Mass properties estimated/1 -> Surfaces UKF estimator/11(Mass_prop_est), Est Mass props/1
  All meas/1 -> Bus Selector1/1, Bus Selector2/1
  Control Eff/1 -> Surfaces UKF estimator/10(Ctrl_effectiveness)
  Control comms/1 -> Surfaces UKF estimator/9(Control_def)
  Bus Selector1/1 -> Surfaces UKF estimator/4(Alt)  "<Alt meas (m)>"
  Bus Selector1/2 -> Surfaces UKF estimator/5(TAS)  "<V_TAS (m/s)>"
  Bus Selector1/3 -> Surfaces UKF estimator/6(AoA)  "<AoA meas (rad)>"
  Bus Selector1/4 -> Surfaces UKF estimator/7(SS)  "<SS meas (rad)>"
  Bus Selector1/5 -> Surfaces UKF estimator/8(omega_b)  "<omega_b meas (rad/s)>"
  Surfaces UKF estimator/2(S_l) -> Mux/1
  Surfaces UKF estimator/3(S_r) -> Mux/2
  Surfaces UKF estimator/4(S_f) -> Mux/3
  Mux/1 -> Memory1/1, To Workspace/1, Est Surfs/1, Demux/1
  Surfaces UKF estimator/1(P_out) -> To Workspace1/1, Memory/1, Determinant of 3x3 Matrix/1
  NO-deviations from base-line model/1 -> Surfaces UKF estimator/12(Deltas_Aero), Est Aero changes/1
  Memory/1 -> Surfaces UKF estimator/1(P)
  Memory1/1 -> Surfaces UKF estimator/2(X_ant)
  Bus Selector2/1 -> Derivative/1  "<omega_b meas (rad/s)>"
  Derivative/1 -> To Workspace2/1, Scope1/1, Surfaces UKF estimator/3(Meas)
  Demux/1 -> Mux1/1  "Left_wing"
  Demux/2 -> Mux1/2  "Right_wing"
  Demux/3 -> Mux1/3  "Fin"
  Mux1/1 -> Scope/1
  Determinant of 3x3 Matrix/1 -> Scope2/1

== system F16ASYM_Controlled/Sensors and filtering/Sensors and filtering. Noise/1st order model1 ==
  y_in : Inport
  Add : Sum  Inputs=|+-
  Integrator : Integrator  InitialCondition=y_i
  K_ref : Gain  Gain=K_ref
  y_out : Outport
  wires:
  y_in/1 -> Add/1
  Add/1 -> K_ref/1
  K_ref/1 -> Integrator/1
  Integrator/1 -> y_out/1, Add/2

== system F16ASYM_Controlled/Sensors and filtering/Sensors and filtering. Noise/1st order model2 ==
  y_in : Inport
  Add : Sum  Inputs=|+-
  Integrator : Integrator  InitialCondition=y_i
  K_ref : Gain  Gain=K_ref
  y_out : Outport
  wires:
  Integrator/1 -> Add/2, y_out/1
  K_ref/1 -> Integrator/1
  Add/1 -> K_ref/1
  y_in/1 -> Add/1

== system F16ASYM_Controlled/Sensors and filtering/Sensors and filtering. Noise/1st order model3 ==
  y_in : Inport
  Add : Sum  Inputs=|+-
  Integrator : Integrator  InitialCondition=y_i
  K_ref : Gain  Gain=K_ref
  y_out : Outport
  wires:
  y_in/1 -> Add/1
  Add/1 -> K_ref/1
  K_ref/1 -> Integrator/1
  Integrator/1 -> y_out/1, Add/2

== system F16ASYM_Controlled/Sensors and filtering/Sensors and filtering. Noise/Inertial Measurement Unit ==
  real angular rate : Inport
  real acceleration : Inport  Port=2
  Add : Sum
  Demux : Demux  Outputs=3
  Mux : Mux  Inputs=3
  Noise : UniformRandomNumber  Minimum=-GYRO.noise_pith  Maximum=GYRO.noise_pith  Seed=346  SampleTime=T_sim
  Noise1 : UniformRandomNumber  Minimum=-ACCEL.noise  Maximum=ACCEL.noise  Seed=134  SampleTime=T_sim
  Noise2 : UniformRandomNumber  Minimum=-GYRO.noise_roll  Maximum=GYRO.noise_roll  Seed=98  SampleTime=T_sim
  Sum{,1..6} (7 alike) : Sum  Inputs=|++
  bias : RandomNumber  Variance=GYRO.bias_repeat  Seed=245  SampleTime=T_sim
  bias1 : RandomNumber  Variance=ACCEL.bias_repeat  Seed=43  SampleTime=T_sim
  bias2 : RandomNumber  Variance=ACCEL.bias_stability  Seed=472  SampleTime=T_sim
  bias3 : RandomNumber  Variance=GYRO.bias_stability  Seed=734  SampleTime=T_sim
  measured angular rate : Outport
  measured acceleration : Outport  Port=2
  wires:
  real acceleration/1 -> Sum/1
  real angular rate/1 -> Sum1/1
  Sum1/1 -> Sum2/1
  Mux/1 -> measured angular rate/1
  Sum/1 -> Sum3/1
  Sum3/1 -> Sum4/1
  Sum4/1 -> measured acceleration/1
  bias1/1 -> Sum/2
  bias2/1 -> Sum3/2
  Noise1/1 -> Sum4/2
  Sum2/1 -> Demux/1
  bias3/1 -> Sum2/2
  bias/1 -> Sum1/2
  Demux/2 -> Sum5/1
  Noise/1 -> Sum5/2, Sum6/2
  Demux/3 -> Sum6/1
  Sum6/1 -> Mux/3
  Sum5/1 -> Mux/2
  Noise2/1 -> Add/1
  Demux/1 -> Add/2
  Add/1 -> Mux/1

== system F16ASYM_Controlled/Stall protection A_z and AoA/AoA and load factor map/If Action Subsystem ==
  Action Port : ActionPort
  From Multimedia File : dspvision/From Multimedia File  inputFilename=C:\Users\David\Documents\Estudios y formación academica\Cranfield\Thesis F16\Work\Solutions\7dof Development\Used Functions\Stall_warning.mp3  loop=on  numPlays=inf  outputStreams=Audio only  videoDataType=single  audioDataType=int16  inheritSampleTime=off  userDefinedSampleTime=T_sim  noAudioOutput=off  isIntensityVideo=off  fourcc=RGB  colorVideoFormat=Separate color signals  outputEOF=off  dataOrg=Column-major  audioFrameSize=1024  computeAudioFrameSize=off  outSamplingMode=Frame based
  To Audio Device : dspsnks4/To Audio Device  deviceName=Default  inheritSampleRate=on  sampleRate=44100  deviceDatatype=Determine from input data type  autoBufferSize=on  bufferSize=4096  queueDuration=1.0
  wires:
  From Multimedia File/1 -> To Audio Device/1

== system F16ASYM_Controlled/Stall protection A_z and AoA/Using AoA/Prediction ==
  V_TAS : Inport
  Add : Sum
  Derivative : Derivative  CoefficientInTFapproximation=1
  T_pred : Gain  Gain=T_pred
  V_tas pred : Outport
  wires:
  V_TAS/1 -> Add/1, Derivative/1
  Derivative/1 -> T_pred/1
  T_pred/1 -> Add/2
  Add/1 -> V_tas pred/1

== system F16ASYM_Controlled/Stall protection A_z and AoA/Using AoA/Sound player ==
  Stall warning : Inport
  Throttle : Inport  Port=2
  Add3 : Sum  OutDataTypeStr=int16  SampleTime=2*T_sim
  Divide : Product  Inputs=**  OutDataTypeStr=int16  SampleTime=2*T_sim
  From Multimedia File : dspvision/From Multimedia File  inputFilename=C:\Users\David\Documents\Estudios y formación academica\Cranfield\Thesis F16\Work\Solutions\7dof Development\Used Functions\Sounds\exhaust_loop.wav  loop=on  numPlays=inf  outputStreams=Audio only  videoDataType=single  audioDataType=int16  inheritSampleTime=off  userDefinedSampleTime=2*T_sim  noAudioOutput=off  isIntensityVideo=off  fourcc=RGB  colorVideoFormat=Separate color signals  outputEOF=off  dataOrg=Column-major  audioFrameSize=1024  computeAudioFrameSize=off  outSamplingMode=Sample based
  Gain1 : Gain  Gain=1/4  OutDataTypeStr=int16
  Gain2 : Gain  Gain=3/4  OutDataTypeStr=int16
  To Audio Device : dspsnks4/To Audio Device  deviceName=Default  inheritSampleRate=on  sampleRate=44100  deviceDatatype=16-bit integer  autoBufferSize=on  bufferSize=4096  queueDuration=4.0  defaultOutputChannelMapping=on  outputChannelMapping=1:2  outputNumUnderrunSamples=off
  wires:
  From Multimedia File/1 -> Divide/1
  Throttle/1 -> Divide/2
  Divide/1 -> Gain1/1
  Stall warning/1 -> Gain2/1
  Add3/1 -> To Audio Device/1
  Gain1/1 -> Add3/2
  Gain2/1 -> Add3/1

== system F16ASYM_Controlled/Stall protection A_z and AoA/Using AoA/Speed stall logic ==
  stall signal : Inport
  Clock : Clock
  Constant : Constant  Value=-0.5/5  SampleTime=T_sim
  Constant1 : Constant  Value=0
  Discrete-Time Integrator : DiscreteIntegrator  ExternalReset=rising  InitialCondition=1  SampleTime=T_sim  LimitOutput=on  UpperSaturationLimit=1  LowerSaturationLimit=0
  pusher : Switch  Threshold=11
  timered signal : Outport
  wires:
  stall signal/1 -> Discrete-Time Integrator/2
  Constant/1 -> Discrete-Time Integrator/1
  Discrete-Time Integrator/1 -> pusher/1
  pusher/1 -> timered signal/1
  Clock/1 -> pusher/2
  Constant1/1 -> pusher/3

== system F16ASYM_Controlled/Stall protection A_z and AoA/Using AoA/Timer signal ==
  Triger : Inport
  Clock : Clock
  Constant : Constant  Value=-1/time_delay
  Constant1 : Constant  Value=0
  Integrator Limited : Integrator  ExternalReset=rising  InitialCondition=1  LimitOutput=on  UpperSaturationLimit=1  LowerSaturationLimit=0
  Relational Operator : RelationalOperator  Operator=~=  OutDataTypeStr=boolean
  pusher : Switch  Threshold=time_delay+1
  Logic output : Outport
  wires:
  Relational Operator/1 -> Logic output/1
  pusher/1 -> Relational Operator/1
  Integrator Limited/1 -> pusher/1
  Clock/1 -> pusher/2
  Constant1/1 -> pusher/3, Relational Operator/2
  Triger/1 -> Integrator Limited/2
  Constant/1 -> Integrator Limited/1

== system F16ASYM_Controlled/Stall protection A_z and AoA/Using AoA/play stall warning ==
  Action Port : ActionPort  InitializeStates=reset  ActionType=then
  From Multimedia File : dspvision/From Multimedia File  inputFilename=C:\Users\David\Documents\Estudios y formación academica\Cranfield\Thesis F16\Work\Solutions\7dof Development\Used Functions\Sounds\Stall_warning.mp3  loop=on  numPlays=inf  outputStreams=Audio only  videoDataType=single  audioDataType=int16  inheritSampleTime=off  userDefinedSampleTime=2*T_sim  noAudioOutput=off  isIntensityVideo=off  fourcc=RGB  colorVideoFormat=Separate color signals  outputEOF=off  dataOrg=Column-major  audioFrameSize=1024  computeAudioFrameSize=off  outSamplingMode=Frame based
  To Audio Device : dspsnks4/To Audio Device  deviceName=Default  inheritSampleRate=on  sampleRate=44100  deviceDatatype=Determine from input data type  autoBufferSize=on  bufferSize=4096  queueDuration=4.0  defaultOutputChannelMapping=on  outputChannelMapping=1:2  outputNumUnderrunSamples=off
  Out1 : Outport
  wires:
  From Multimedia File/1 -> To Audio Device/1, Out1/1

== system F16ASYM_Controlled/Control allocator/Control allocator: NO RECONF/Leading Edge Flap:Symetric deflection/Creating    qbar // ps ==
  alt : Inport
  V : Inport  Port=2
  ISA Atmosphere Model : aerolibatmos2/ISA Atmosphere Model  custom=off  g=9.80665  gamma=1.4  R=287.0531  L=0.0065  h_trop=11000  h_strat=20000  rho0=1.225  P0=101325  T0=288.15  h0=0
  Math Function1 : Math  Operator=square  SaturateOnIntegerOverflow=on
  Product : Product  Inputs=/*  SaturateOnIntegerOverflow=on  InputSameDT=on  OutDataTypeStr=Inherit: Same as first input
  Product5 : Product  Inputs=**  SaturateOnIntegerOverflow=on  InputSameDT=on  OutDataTypeStr=Inherit: Same as first input
  Terminator : Terminator
  Terminator1 : Terminator
  r2d4 : Gain  Gain=0.5  SaturateOnIntegerOverflow=on  OutDataTypeStr=Inherit: Same as input  ParamDataTypeStr=Inherit: Same as input
  qbar / ps : Outport
  wires:
  ISA Atmosphere Model/2 -> Terminator1/1
  ISA Atmosphere Model/1 -> Terminator/1
  ISA Atmosphere Model/3 -> Product/1
  ISA Atmosphere Model/4 -> Product5/1
  Product/1 -> qbar / ps/1
  V/1 -> Math Function1/1
  Product5/1 -> Product/2  "qbar"
  r2d4/1 -> Product5/2
  Math Function1/1 -> r2d4/1
  alt/1 -> ISA Atmosphere Model/1

== system F16ASYM_Controlled/Control allocator/Control allocator: RECONFIG/Blockades logic: Limits injetor/1st order model ==
  y_in : Inport
  Add : Sum  Inputs=|+-
  Integrator : Integrator  InitialCondition=y_i
  K_ref : Gain  Gain=K_ref
  y_out : Outport
  wires:
  Integrator/1 -> Add/2, y_out/1
  K_ref/1 -> Integrator/1
  Add/1 -> K_ref/1
  y_in/1 -> Add/1

== system F16ASYM_Controlled/Control allocator/Control allocator: RECONFIG/Blockades logic: Limits injetor/1st order model1 ==
  y_in : Inport
  Add : Sum  Inputs=|+-
  Integrator : Integrator  InitialCondition=y_i
  K_ref : Gain  Gain=K_ref
  y_out : Outport
  wires:
  y_in/1 -> Add/1
  Add/1 -> K_ref/1
  K_ref/1 -> Integrator/1
  Integrator/1 -> y_out/1, Add/2

== system F16ASYM_Controlled/Control allocator/Control allocator: RECONFIG/Blockades logic: Limits injetor/Block AT INFERIOR LIMIT ==
  Limit : Inport
  Blockades : Inport  Port=2
  Demux : Demux  Outputs=7
  Logical Operator : Logic  Operator=NOT  IconShape=distinctive  AllPortsSameDT=off  OutDataTypeStr=boolean
  Mux1 : Mux  Inputs=7
  Mux2 : Mux  Inputs=7
  Selector : Selector  InputPortWidth=7
  Selector1 : Selector  InputPortWidth=7  Indices=2
  Selector2 : Selector  InputPortWidth=7  Indices=3
  Selector3 : Selector  InputPortWidth=7  Indices=4
  Selector4 : Selector  InputPortWidth=7  Indices=5
  Selector5 : Selector  InputPortWidth=7  Indices=6
  Selector6 : Selector  InputPortWidth=7  Indices=7
  Switch{,1..6} (7 alike) : Switch  Threshold=0.5
  isNaN{,1..6} (7 alike) : RelationalOperator  Operator=isNaN  OutDataTypeStr=boolean
  Reconfig limits : Outport
  Surf blocked : Outport  Port=2
  wires:
  [Blockades] -> Selector/1
  isNaN/1 -> [left_elev], Switch/2
  Demux/1 -> Switch/1
  Selector/1 -> Switch/3, isNaN/1
  [Blockades] -> Selector1/1
  isNaN1/1 -> [right_elev], Switch1/2
  Demux/2 -> Switch1/1
  Selector1/1 -> Switch1/3, isNaN1/1
  [Blockades] -> Selector2/1
  isNaN2/1 -> Switch2/2, [left_ail]
  Demux/3 -> Switch2/1
  Selector2/1 -> Switch2/3, isNaN2/1
  [Blockades] -> Selector3/1
  isNaN3/1 -> [right_ail], Switch3/2
  Demux/4 -> Switch3/1
  Selector3/1 -> Switch3/3, isNaN3/1
  [Blockades] -> Selector4/1
  isNaN4/1 -> [rudder], Switch4/2
  Demux/5 -> Switch4/1
  Selector4/1 -> Switch4/3, isNaN4/1
  [Blockades] -> Selector5/1
  isNaN5/1 -> [left_LEF], Switch5/2
  Demux/6 -> Switch5/1
  Selector5/1 -> Switch5/3, isNaN5/1
  [Blockades] -> Selector6/1
  isNaN6/1 -> [rith_LEF], Switch6/2
  Demux/7 -> Switch6/1
  Selector6/1 -> Switch6/3, isNaN6/1
  Limit/1 -> Demux/1
  Mux2/1 -> Reconfig limits/1
  Blockades/1 -> [Blockades]
  Switch/1 -> Mux2/1  "Elevator_L"
  Switch1/1 -> Mux2/2
  Switch2/1 -> Mux2/3  "Aileron_L"
  Switch3/1 -> Mux2/4  "Aileron_R"
  Switch4/1 -> Mux2/5  "Rudder"
  Switch5/1 -> Mux2/6  "LEF_L"
  Switch6/1 -> Mux2/7
  [left_elev] -> Mux1/1
  Mux1/1 -> Logical Operator/1
  [right_elev] -> Mux1/2
  [left_ail] -> Mux1/3
  [right_ail] -> Mux1/4
  [rudder] -> Mux1/5
  [left_LEF] -> Mux1/6
  [rith_LEF] -> Mux1/7
  Logical Operator/1 -> Surf blocked/1
